simulink model "vehicle_sim"  (R2024b)
settings: Solver=VariableStepAuto  StartTime=0.0  StopTime=4  RelTol=1e-3
libraries: inverter_model x4, tire_model x4, vehdynlibsteering x1, autolibshared x1, vehdynlibviscommon x1, battery x1
settings Model: Creator=jessi  LastModifiedBy=jessi

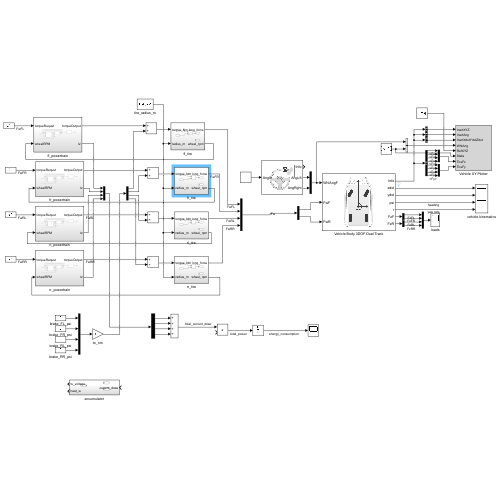
[thumbnail: Simulink's stored preview of the top-level diagram]
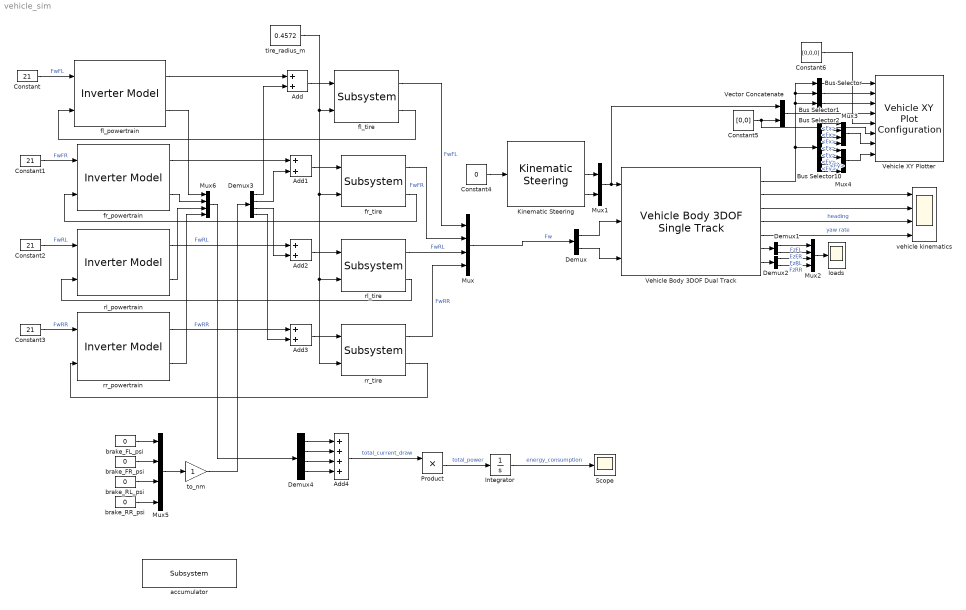
== system vehicle_sim ==
  Add{,1..3} (4 alike) : Sum
  Add4 : Sum  Inputs=++++
  Bus Selector : BusSelector  OutputSignals=InertFrm.Cg.Disp.X,InertFrm.Cg.Disp.Y,InertFrm.Cg.Disp.Z  OutputAsBus=on
  Bus Selector1 : BusSelector  OutputSignals=InertFrm.Cg.Ang.phi,InertFrm.Cg.Ang.theta,InertFrm.Cg.Ang.psi  OutputAsBus=on
  Bus Selector10 : BusSelector  OutputSignals=BdyFrm.Forces.Tires.FrntTires.Lft.Fx,BdyFrm.Forces.Tires.FrntTires.Rght.Fx,BdyFrm.Forces.Tires.RearTires.Lft.Fx,BdyFrm.Forces.Tires.RearTires.Rght.Fx,BdyFrm.Forces.Tires.FrntTires.Lft.Fy,BdyFrm.Forces.Tires.FrntTires.Rght.Fy,BdyFrm.Forces.Tires.RearTires.Lft.Fy,BdyFrm.Forces.Tires.RearTires.Rght.Fy
  Bus Selector2 : BusSelector  OutputSignals=InertFrm.Cg.Vel.Xdot,InertFrm.Cg.Vel.Ydot,InertFrm.Cg.Vel.Zdot  OutputAsBus=on
  Constant{,1..3} (4 alike) : Constant  Value=21
  Constant4 : Constant  Value=0
  Constant5 : Constant  Value=[0,0]
  Constant6 : Constant  Value=[0,0,0]
  Demux : Demux  Outputs=2
  Demux1 : Demux  Outputs=2
  Demux2 : Demux  Outputs=2
  Demux3 : Demux
  Demux4 : Demux
  Integrator : Integrator
  Kinematic Steering : vehdynlibsteering/Kinematic Steering  StrgType=Rack and pinion  StrgRatioType=Constant  Loc=Front  NrmlFctr=0.01  TrckWdth=1  WhlBase=1.524  Db=0  StrgRng=1.25*pi  StrgAngBpts="[-6.2832   -5.0265   -3.7699   -2.5133   -1.2566         0    1.2566    2.5133    3.7699    5.0265    6.2832]"  StrgRatioTbl=|  StrgRatio=100  PctAckIn=off  PctAck=100  PctAckTbl=ones(1,11)*100  StrgArmLngth=0.1  RckCsLngth=0.5  TieRodLngth=0.248  D=0.2  PnnRadius=0.00085818  PnnRadiusTbl="[0.0055    0.0055    0.0056    0.0057    0.0058    0.0057    0.0057    0.0057    0.0056    0.0055    0.0055]"  RodLngth=0.1  ParaArmLngth=0.9  aMode=2
      | [13.5000   13.3750   13.2500   13.1250   13.0000   13.0000   13.0000   13.1250   13.2500   13.3750   13.5000
      | ]
  Mux{,2..6} (6 alike) : Mux
  Mux1 : Mux  Inputs=2
  Product : Product
  Scope : Scope
  Vector Concatenate : Concatenate
  Vehicle Body 3DOF Dual Track : autolibshared/Vehicle Body 3DOF Single Track  trackMode=Dual  inputMode=External longitudinal forces  frontSteerMode=on  rearSteerMode=off  windMode=off  muMode=off  extFMode=off  extMMode=off  htchFMode=off  htchMMode=off  extXo=off  extpsio=off  extxdoto=off  extro=off  extYo=off  extTamb=off  extydoto=off  aMode=2  NF=2  NR=2  m=300  a=0.837  b=0.713  h=0.30  dh=1  hh=0.2  X_o=0  xdot_o=0  CalphaMode=off  sigmaMode=on  d=0  hl=0  w=[1.1,1.1]  Cy_f=12e3  Cy_r=11e3  sigma_f=.1  sigma_r=.1  alpha_f_brk=[-.1 .1]  Cy_f_data=[-9e3 9e3]  alpha_r_brk=[-.1 .1]  Cy_r_data=[-9e3 9e3]  Y_o=0  ydot_o=0  Izz=4000  psi_o=0  r_o=0  Af=2  Cd=.3  Cl=.1  Cpm=.1  beta_w=[0 0.01:0.01:0.3]  Cs=[0:0.03:0.9]  Cym=[0 1e-6:0.01:0.3]  Pabs=101325  Tair=303  g=9.81  mu=1  xdot_tol=.01  Fznom=1961  Fxtire_sat=7e4  Fytire_sat=7e4  longOff=0  latOff=0  vertOff=0  wrapAng=off
      settings: LibrarySourceBlock=vehdynlibeom/Vehicle Body 3DOF Dual Track
  Vehicle XY Plotter : vehdynlibviscommon/Vehicle XY Plot Configuration  extRef=on  extStats=on  extTireF=on  a=0.837  b=0.713  w=1.1  figBorder=10  bufferSize=2048  velNorm=10  tireFNorm=100  pltDT=.2
  accumulator : battery/Subsystem  SystemSampleTime=-1  VariantActivationTime=update diagram  AllowFlexibleInterface=on  Latency=0  AutoFrameSizeCalculation=off
  brake_FL_psi : Constant  Value=0
  brake_FR_psi : Constant  Value=0
  brake_RL_psi : Constant  Value=0
  brake_RR_psi : Constant  Value=0
  fl_powertrain : inverter_model/Inverter Model  SystemSampleTime=-1  VariantActivationTime=update diagram  AllowFlexibleInterface=on  Latency=0  AutoFrameSizeCalculation=off
  fl_tire : tire_model/Subsystem  SystemSampleTime=-1  VariantActivationTime=update diagram  AllowFlexibleInterface=on  Latency=0  AutoFrameSizeCalculation=off
  fr_powertrain : inverter_model/Inverter Model  SystemSampleTime=-1  VariantActivationTime=update diagram  AllowFlexibleInterface=on  Latency=0  AutoFrameSizeCalculation=off
  fr_tire : tire_model/Subsystem  SystemSampleTime=-1  VariantActivationTime=update diagram  AllowFlexibleInterface=on  Latency=0  AutoFrameSizeCalculation=off
  loads : Scope
  rl_powertrain : inverter_model/Inverter Model  SystemSampleTime=-1  VariantActivationTime=update diagram  AllowFlexibleInterface=on  Latency=0  AutoFrameSizeCalculation=off
  rl_tire : tire_model/Subsystem  SystemSampleTime=-1  VariantActivationTime=update diagram  AllowFlexibleInterface=on  Latency=0  AutoFrameSizeCalculation=off
  rr_powertrain : inverter_model/Inverter Model  SystemSampleTime=-1  VariantActivationTime=update diagram  AllowFlexibleInterface=on  Latency=0  AutoFrameSizeCalculation=off
  rr_tire : tire_model/Subsystem  SystemSampleTime=-1  VariantActivationTime=update diagram  AllowFlexibleInterface=on  Latency=0  AutoFrameSizeCalculation=off
  tire_radius_m : Constant  Value=0.4572
  to_nm : Gain
  vehicle kinematics : Scope  NumInputPorts=4
  wires:
  Demux/1 -> Vehicle Body 3DOF Dual Track/2
  fl_tire/1 -> Mux/1  "FwFL"
  fr_powertrain/1 -> Add1/1
  rl_tire/1 -> Mux/3  "FwRL"
  rr_tire/1 -> Mux/4  "FwRR"
  Mux/1 -> Demux/1  "Fw"
  Demux/2 -> Vehicle Body 3DOF Dual Track/3
  Vehicle Body 3DOF Dual Track/2 -> vehicle kinematics/1
  Vehicle Body 3DOF Dual Track/3 -> vehicle kinematics/2
  Vehicle Body 3DOF Dual Track/4 -> vehicle kinematics/3  "heading"
  Vehicle Body 3DOF Dual Track/5 -> vehicle kinematics/4  "yaw rate"
  Kinematic Steering/2 -> Mux1/1
  Kinematic Steering/3 -> Mux1/2
  Mux1/1 -> Vector Concatenate/1, Vehicle Body 3DOF Dual Track/1
  Constant4/1 -> Kinematic Steering/1
  Vehicle Body 3DOF Dual Track/6 -> Demux1/1
  Vehicle Body 3DOF Dual Track/7 -> Demux2/1
  Demux1/1 -> Mux2/1  "FzFL"
  Demux1/2 -> Mux2/2  "FzFR"
  Demux2/1 -> Mux2/3  "FzRL"
  Demux2/2 -> Mux2/4  "FzRR"
  Mux2/1 -> loads/1
  Constant/1 -> fl_powertrain/1  "FwFL"
  Constant1/1 -> fr_powertrain/1  "FwFR"
  Constant2/1 -> rl_powertrain/1  "FwRL"
  Constant3/1 -> rr_powertrain/1  "FwRR"
  fl_powertrain/1 -> Add/1
  fr_tire/1 -> Mux/2  "FwFR"
  rr_powertrain/1 -> Add3/1  "FwRR"
  rl_powertrain/1 -> Add2/1  "FwRL"
  tire_radius_m/1 -> fl_tire/2, fr_tire/2, rl_tire/2, rr_tire/2
  Vehicle Body 3DOF Dual Track/1 -> Bus Selector2/1, Bus Selector/1, Bus Selector1/1, Bus Selector10/1
  Bus Selector/1 -> Vehicle XY Plotter/1
  Bus Selector1/1 -> Vehicle XY Plotter/2
  Bus Selector2/1 -> Vehicle XY Plotter/3
  Bus Selector10/1 -> Mux3/1  "<Fx>"
  Bus Selector10/2 -> Mux3/2  "<Fx>"
  Bus Selector10/3 -> Mux3/3  "<Fx>"
  Bus Selector10/4 -> Mux3/4  "<Fx>"
  Bus Selector10/5 -> Mux4/1  "<Fy>"
  Bus Selector10/6 -> Mux4/2  "<Fy>"
  Bus Selector10/7 -> Mux4/3  "<Fy>"
  Bus Selector10/8 -> Mux4/4  "<Fy>"
  Mux3/1 -> Vehicle XY Plotter/7
  Mux4/1 -> Vehicle XY Plotter/8
  Constant5/1 -> Vehicle XY Plotter/6, Vector Concatenate/2
  Vector Concatenate/1 -> Vehicle XY Plotter/4
  Constant6/1 -> Vehicle XY Plotter/5
  brake_FL_psi/1 -> Mux5/1
  brake_FR_psi/1 -> Mux5/2
  brake_RL_psi/1 -> Mux5/3
  brake_RR_psi/1 -> Mux5/4
  Mux5/1 -> to_nm/1
  Add/1 -> fl_tire/1
  Add2/1 -> rl_tire/1
  Add1/1 -> fr_tire/1
  Add3/1 -> rr_tire/1
  Add4/1 -> Product/1  "total_current_draw"
  to_nm/1 -> Demux3/1
  Integrator/1 -> Scope/1  "energy_consumption"
  Product/1 -> Integrator/1  "total_power"
  fl_tire/2 -> fl_powertrain/2
  fr_tire/2 -> fr_powertrain/2
  rl_tire/2 -> rl_powertrain/2
  rr_tire/2 -> rr_powertrain/2
  Demux3/1 -> Add/2
  Demux3/2 -> Add1/2
  Demux3/3 -> Add2/2
  Demux3/4 -> Add3/2
  fl_powertrain/2 -> Mux6/1
  fr_powertrain/2 -> Mux6/2
  rl_powertrain/2 -> Mux6/3
  rr_powertrain/2 -> Mux6/4
  Demux4/1 -> Add4/1
  Demux4/2 -> Add4/2
  Demux4/3 -> Add4/3
  Demux4/4 -> Add4/4
  Mux6/1 -> Demux4/1
